simulink model "sampleModel174"  (R2021b)
settings: Solver=VariableStepAuto  StartTime=0.0  StopTime=10.0  RelTol=1e-3
undefined symbols (not defined in the file or in its folder): Newton, Raphson
libraries: simulink x7
settings Model: Creator=user  LastModifiedBy=user

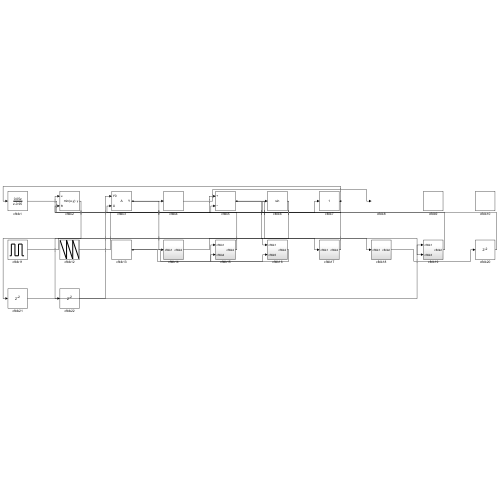
[thumbnail: Simulink's stored preview of the top-level diagram]
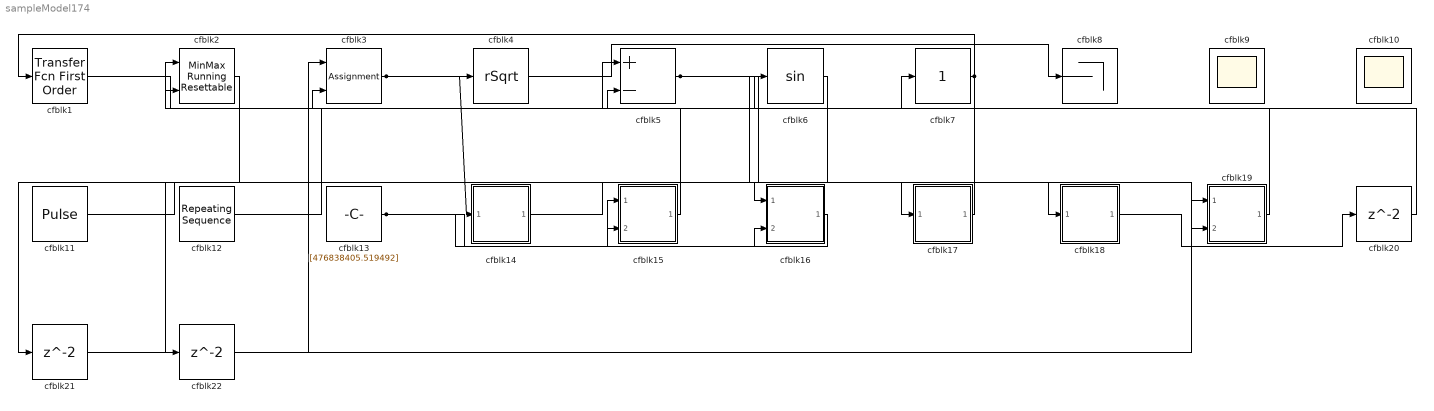
== system sampleModel174 ==
  cfblk1 : simulink/Discrete/Transfer Fcn First Order  PoleZ=0.95  ICPrevOutput=0.0  DoSatur=off
  cfblk10 : Scope
      settings: Floating=on
  cfblk11 : DiscretePulseGenerator  PulseType=Time based  Amplitude=[-279898301.417747]  Period=[25568110.472088]  PulseWidth=5  PhaseDelay=[7.000000]
  cfblk12 : simulink/Sources/Repeating Sequence  rep_seq_t=[0 2]  rep_seq_y=[242561197.518301, -428068926.056757]
  cfblk13 : Constant  Value=[476838405.519492]  SampleTime=1
  cfblk14 : Subsystem
  cfblk15 : Subsystem
  cfblk16 : Subsystem
  cfblk17 : Subsystem
  cfblk18 : Subsystem
  cfblk19 : Subsystem
  cfblk2 : simulink/Math Operations/MinMax Running Resettable  Function=min  vinit=0.0
  cfblk20 : Delay  SampleTime=1
  cfblk21 : Delay  SampleTime=1
  cfblk22 : Delay  SampleTime=1
  cfblk3 : Assignment  DiagnosticForDimensions=Warning  IndexOptions=Index vector (dialog)  Indices=1  OutputSizes=1
  cfblk4 : Sqrt  Operator=rSqrt  AlgorithmType=Newton-Raphson  SaturateOnIntegerOverflow=on
  cfblk5 : Sum  Inputs=+-
  cfblk6 : Trigonometry
  cfblk7 : simulink/Math Operations/Slider Gain  gain=1  low=0  high=2
  cfblk8 : Terminator
  cfblk9 : Scope
      settings: Floating=on
  wires:
  cfblk19/1(cfblk2) -> cfblk2/1
  cfblk5/1 -> cfblk18/1(cfblk1), cfblk19/2(cfblk3)
  cfblk7/1 -> cfblk1/1, cfblk3/2
  cfblk17/1(cfblk2) -> cfblk6/1
  cfblk4/1 -> cfblk8/1
  cfblk11/1 -> cfblk16/1(cfblk1)
  cfblk13/1 -> cfblk15/1(cfblk1), cfblk16/2(cfblk5)
  cfblk12/1 -> cfblk7/1
  cfblk1/1 -> cfblk5/2
  cfblk16/1(cfblk2) -> cfblk15/2(cfblk4)
  cfblk14/1(cfblk2) -> cfblk17/1(cfblk1)
  cfblk3/1 -> cfblk14/1(cfblk1), cfblk4/1
  cfblk15/1(cfblk2) -> cfblk2/2
  cfblk18/1(cfblk2) -> cfblk20/1
  cfblk20/1 -> cfblk5/1
  cfblk2/1 -> cfblk21/1
  cfblk21/1 -> cfblk19/1(cfblk1)
  cfblk6/1 -> cfblk22/1
  cfblk22/1 -> cfblk3/1

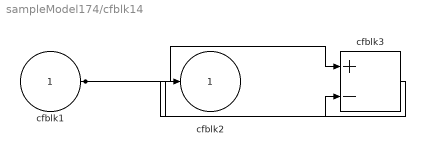
== system sampleModel174/cfblk14 ==
  cfblk1 : Inport
  cfblk3 : Sum  Inputs=+-
  cfblk2 : Outport
  wires:
  cfblk1/1 -> cfblk3/1, cfblk3/2
  cfblk3/1 -> cfblk2/1

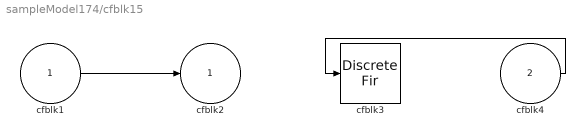
== system sampleModel174/cfblk15 ==
  cfblk1 : Inport
  cfblk4 : Inport  Port=2
  cfblk3 : DiscreteFir  SampleTime=1
  cfblk2 : Outport
  wires:
  cfblk4/1 -> cfblk3/1
  cfblk1/1 -> cfblk2/1

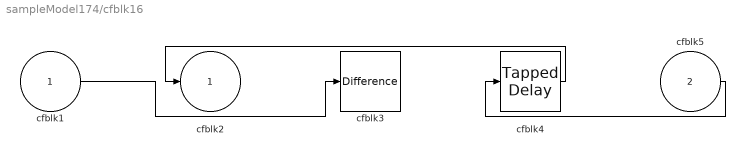
== system sampleModel174/cfblk16 ==
  cfblk1 : Inport
  cfblk5 : Inport  Port=2
  cfblk3 : simulink/Discrete/Difference  ICPrevInput=0.0  OutMin=[]  OutMax=[]  OutDataTypeStr=Inherit: Inherit via back propagation  OutDataType=fixdt(1, 16)  OutScaling=2^-10  DoSatur=off
  cfblk4 : simulink/Discrete/Tapped Delay  vinit=0.0  samptime=-1  NumDelays=1  DelayOrder=Oldest  includeCurrent=off
  cfblk2 : Outport
  wires:
  cfblk4/1 -> cfblk2/1
  cfblk1/1 -> cfblk3/1
  cfblk5/1 -> cfblk4/1

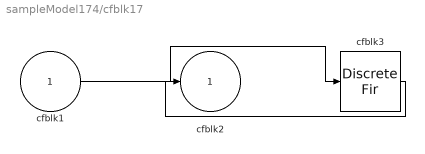
== system sampleModel174/cfblk17 ==
  cfblk1 : Inport
  cfblk3 : DiscreteFir  SampleTime=1
  cfblk2 : Outport
  wires:
  cfblk1/1 -> cfblk3/1
  cfblk3/1 -> cfblk2/1

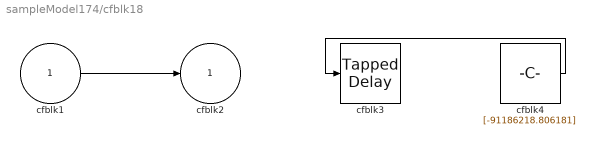
== system sampleModel174/cfblk18 ==
  cfblk1 : Inport
  cfblk3 : simulink/Discrete/Tapped Delay  vinit=0.0  samptime=-1  NumDelays=1  DelayOrder=Oldest  includeCurrent=off
  cfblk4 : Constant  Value=[-91186218.806181]  SampleTime=1
  cfblk2 : Outport
  wires:
  cfblk4/1 -> cfblk3/1
  cfblk1/1 -> cfblk2/1

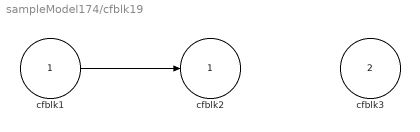
== system sampleModel174/cfblk19 ==
  cfblk1 : Inport
  cfblk3 : Inport  Port=2
  cfblk2 : Outport
  wires:
  cfblk1/1 -> cfblk2/1
